simulink model "shiyan1_1"  (R2021b)
settings: Solver=FixedStepAuto  StartTime=0.0  StopTime=30  FixedStep=0.001  RelTol=1e-3
libraries: simulink x1
settings Model: Creator=Administrator  LastModifiedBy=Administrator

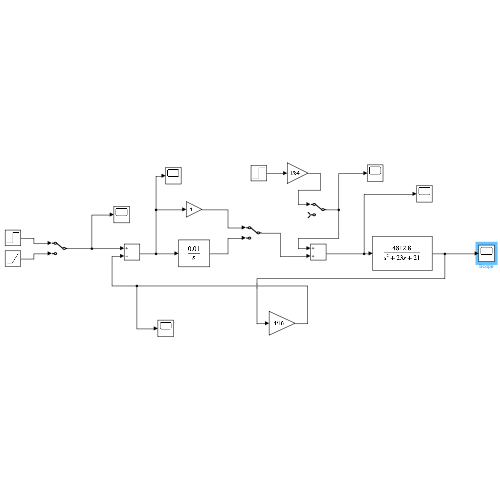
[thumbnail: Simulink's stored preview of the top-level diagram]
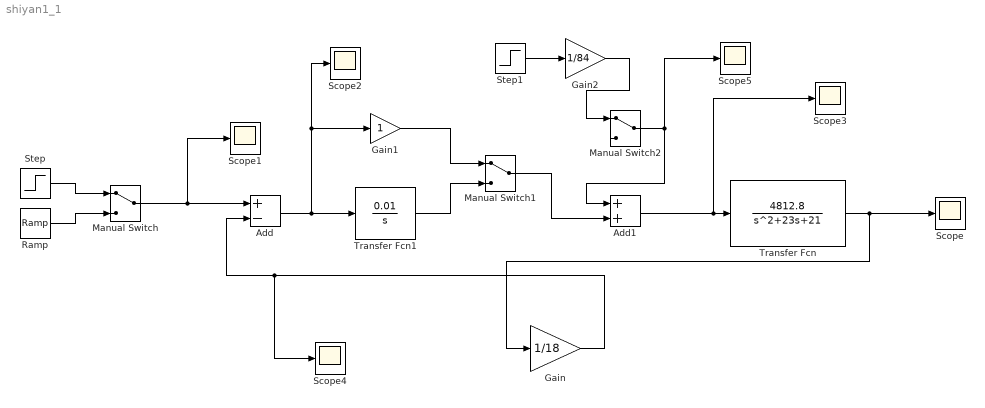
== system shiyan1_1 ==
  Add : Sum  Inputs=+-
  Add1 : Sum
  Gain : Gain  Gain=1/18
  Gain1 : Gain
  Gain2 : Gain  Gain=1/84
  Manual Switch : ManualSwitch
  Manual Switch1 : ManualSwitch
  Manual Switch2 : ManualSwitch
  Ramp : simulink/Sources/Ramp  slope=1  start=0  InitialOutput=0
  Scope{,1..5} (6 alike) : Scope
  Step : Step  SampleTime=0
  Step1 : Step  Time=10  After=17  SampleTime=0
  Transfer Fcn : TransferFcn  Numerator=[4812.8]  Denominator=[1 23 21]
  Transfer Fcn1 : TransferFcn  Numerator=[0.01]  Denominator=[1 0]
  wires:
  Add/1 -> Scope2/1, Gain1/1, Transfer Fcn1/1
  Transfer Fcn/1 -> Gain/1, Scope/1
  Gain/1 -> Add/2, Scope4/1
  Step1/1 -> Gain2/1
  Add1/1 -> Scope3/1, Transfer Fcn/1
  Step/1 -> Manual Switch/1
  Ramp/1 -> Manual Switch/2
  Manual Switch/1 -> Scope1/1, Add/1
  Gain1/1 -> Manual Switch1/1
  Transfer Fcn1/1 -> Manual Switch1/2
  Manual Switch1/1 -> Add1/2
  Gain2/1 -> Manual Switch2/1
  Manual Switch2/1 -> Scope5/1, Add1/1
